simulink model "uuv_depth_control"  (R2021a)
settings: Solver=ode1  StartTime=0  StopTime=1000  FixedStep=0.1  RelTol=1e-3
undefined symbols (not defined in the file or in its folder): sigbuilder_block
(part 1 of 2)
settings Model: NumberOfSteps=10  PacingRate=1000  Creator=53549  LastModifiedBy=21847
settings DataIOCC: ReturnWorkspaceOutputs=off
settings DebuggingCC: SFMachineParentedDataDiag=warning  ArithmeticOperatorsInVariantConditions=warning
settings SFSimCC: SimUseLocalCustomCode=off  CustomCodeUndefinedFunction=UseInterfaceOnly
settings RTWCC: RTWUseLocalCustomCode=off
settings CodeAppCC: StateflowObjectComments=on

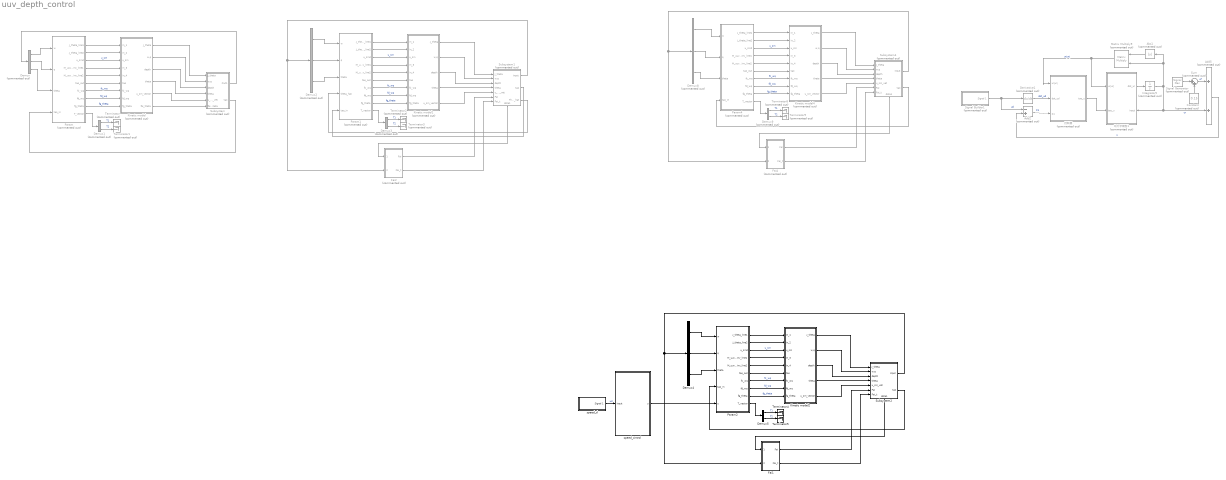
== system uuv_depth_control ==
  Abs1 : Abs  Commented=on
  Add2 : Sum  Commented=on  Inputs=-+
  Add5 : Sum  Commented=on
  Constant : Constant  Commented=on  Value=0.15
  Demux : Demux  Commented=on  Outputs=3
  Demux1 : Demux  Commented=on  Outputs=2
  Demux2 : Demux  Commented=on  Outputs=3
  Demux3 : Demux  Commented=on  Outputs=2
  Demux4 : Demux  Outputs=3
  Demux5 : Demux  Outputs=2
  Demux8 : Demux  Commented=on  Outputs=3
  Demux9 : Demux  Commented=on  Outputs=2
  Derivative1 : Derivative  Commented=on
  Fai1 : Subsystem
  Fai2 : Subsystem  Commented=on
  Fai4 : Subsystem  Commented=on
  Integrator5 : Integrator  Commented=on
  Kinetic model : Subsystem  Commented=on
  Kinetic model1 : Subsystem  Commented=on
  Kinetic model2 : Subsystem
  Kinetic model4 : Subsystem  Commented=on
  Matrix Multiply9 : Product  Commented=on  Multiplication=Matrix(*)
  Param : MATLAB Function  Commented=on  TreatAsAtomicUnit=on
  Param1 : MATLAB Function  Commented=on  TreatAsAtomicUnit=on
  Param2 : MATLAB Function  TreatAsAtomicUnit=on
  Param4 : MATLAB Function  Commented=on  TreatAsAtomicUnit=on
  Signal Generator : SignalGenerator  Commented=on  Amplitude=0.2  Frequency=0.0143
  Signal Builder1 : Subsystem  Tag=STV Subsys  Commented=on  LoadFcn=sigbuilder_block('load');  StartFcn=sigbuilder_block('start');  StopFcn=sigbuilder_block('stop');  ClipboardFcn=sigbuilder_block('clipboard');  mask(Sigbuilder block){tuvar=[0:10]}
      mask help: Simulink:masks:SigbuilderBlock_MD
      mask init:
      | if ~strcmp(get_param(bdroot(gcbh),'SimulationStatus'),'stopped') tuvar = sigbuilder_block('maskInit'); end
      settings: CopyFcn=sigbuilder_block('copy');  DeleteFcn=sigbuilder_block('delete');  ModelCloseFcn=sigbuilder_block('modelClose');  PreSaveFcn=sigbuilder_block('preSave');  PauseFcn=sigbuilder_block('pause');  ContinueFcn=sigbuilder_block('continue');  NameChangeFcn=sigbuilder_block('namechange');  OpenFcn=sigbuilder_block('open',[437.6 199.2 550.4 400 ]);  CloseFcn=sigbuilder_block('close');
      mask Display: plot(0, 0, 100, 100,[2, 2, 32, 32, 2], [68, 8, 8, 68, 68],[32, 2], [38, 38], [32, 19, 2],[53, 60, 44], [32, 17, 17, 2],[16, 16, 31, 31]);txt = getActiveGroup(gcbh);text(2, 100, txt,'verticalAlignment', 'top');
  Subsystem : Subsystem  Commented=on
  Subsystem1 : Subsystem  Commented=on
      settings: PortSchema="{\"entries\":[{\"content\":{\"sides\":[{\"content\":{\"connectorIds\":[\"In1\",\"In2\",\"In3\",\"In4\",\"In5\",\"In6\",\"In7\"]},\"type\":\"ConnectorPlacement.EquallySpacedRectSide\",\"uuid\":\"5c5a44e6-8d8e-440f-9e7c-8dc2648a5aa2\"},{\"content\":{\"connectorIds\":[\"Out1\",\"Out2\",\"Out3\"],\"side\":\"RIGHT\"},\"type\":\"ConnectorPlacement.EquallySpacedRectSide\",\"uuid\":\"bbda16c8-79bf-4e81-8c5f-170a18e1caa9\"},{\"content\":{\"connectorIds\":[],\"side\":\"TOP\"},\"type\":\"ConnectorPlacement.EquallySpacedRectSide\",\"uuid\":\"ec6df362-669b-4b04-85b5-b778e5b376fb\"},{\"content\":{\"connectorIds\":[\"Out4\"],\"side\":\"BOTTOM\"},\"type\":\"ConnectorPlacement.EquallySpacedRectSide\",\"uuid\":\"b375aecc-e755-48ed-98c2-53f6a7777844\"}]},\"type\":\"ConnectorPlacement.EquallySpacedConnector\",\"uuid\":\"a63cd60f-02eb-402d-846a-0ab9a0543d99\"}],\"packageUris\":[\"http://schema.mathworks.com/mf0/Connector/R2020b\"],\"version\":\"1.0\"}"
  Subsystem2 : Subsystem
      settings: PortSchema="{\"entries\":[{\"content\":{\"sides\":[{\"content\":{\"connectorIds\":[\"In1\",\"In2\",\"In3\",\"In4\",\"In5\",\"In6\",\"In7\"]},\"type\":\"ConnectorPlacement.EquallySpacedRectSide\",\"uuid\":\"5c5a44e6-8d8e-440f-9e7c-8dc2648a5aa2\"},{\"content\":{\"connectorIds\":[\"Out1\",\"Out2\"],\"side\":\"RIGHT\"},\"type\":\"ConnectorPlacement.EquallySpacedRectSide\",\"uuid\":\"bbda16c8-79bf-4e81-8c5f-170a18e1caa9\"},{\"content\":{\"connectorIds\":[],\"side\":\"TOP\"},\"type\":\"ConnectorPlacement.EquallySpacedRectSide\",\"uuid\":\"ec6df362-669b-4b04-85b5-b778e5b376fb\"},{\"content\":{\"connectorIds\":[\"Out3\"],\"side\":\"BOTTOM\"},\"type\":\"ConnectorPlacement.EquallySpacedRectSide\",\"uuid\":\"b375aecc-e755-48ed-98c2-53f6a7777844\"}]},\"type\":\"ConnectorPlacement.EquallySpacedConnector\",\"uuid\":\"a63cd60f-02eb-402d-846a-0ab9a0543d99\"}],\"packageUris\":[\"http://schema.mathworks.com/mf0/Connector/R2020b\"],\"version\":\"1.0\"}"
  Subsystem4 : Subsystem  Commented=on
      settings: PortSchema="{\"entries\":[{\"content\":{\"sides\":[{\"content\":{\"connectorIds\":[\"In1\",\"In2\",\"In3\",\"In4\",\"In5\",\"In6\",\"In7\"]},\"type\":\"ConnectorPlacement.EquallySpacedRectSide\",\"uuid\":\"5c5a44e6-8d8e-440f-9e7c-8dc2648a5aa2\"},{\"content\":{\"connectorIds\":[\"Out1\",\"Out2\"],\"side\":\"RIGHT\"},\"type\":\"ConnectorPlacement.EquallySpacedRectSide\",\"uuid\":\"bbda16c8-79bf-4e81-8c5f-170a18e1caa9\"},{\"content\":{\"connectorIds\":[],\"side\":\"TOP\"},\"type\":\"ConnectorPlacement.EquallySpacedRectSide\",\"uuid\":\"ec6df362-669b-4b04-85b5-b778e5b376fb\"},{\"content\":{\"connectorIds\":[\"Out3\"],\"side\":\"BOTTOM\"},\"type\":\"ConnectorPlacement.EquallySpacedRectSide\",\"uuid\":\"b375aecc-e755-48ed-98c2-53f6a7777844\"}]},\"type\":\"ConnectorPlacement.EquallySpacedConnector\",\"uuid\":\"a63cd60f-02eb-402d-846a-0ab9a0543d99\"}],\"packageUris\":[\"http://schema.mathworks.com/mf0/Connector/R2020b\"],\"version\":\"1.0\"}"
  Sum : Sum  Commented=on  Inputs=|++
  Terminator{,1..3,8..9} (6 alike) : Terminator  Commented=on
  Terminator4 : Terminator
  Terminator5 : Terminator
  speed_cintrol : Subsystem
  speed_d : Subsystem  Tag=STV Subsys  LoadFcn=sigbuilder_block('load');  StartFcn=sigbuilder_block('start');  StopFcn=sigbuilder_block('stop');  ClipboardFcn=sigbuilder_block('clipboard');  mask(Sigbuilder block){tuvar=[0:10]}
      mask help: Simulink:masks:SigbuilderBlock_MD
      mask init:
      | if ~strcmp(get_param(bdroot(gcbh),'SimulationStatus'),'stopped') tuvar = sigbuilder_block('maskInit'); end
      settings: CopyFcn=sigbuilder_block('copy');  DeleteFcn=sigbuilder_block('delete');  ModelCloseFcn=sigbuilder_block('modelClose');  PreSaveFcn=sigbuilder_block('preSave');  PauseFcn=sigbuilder_block('pause');  ContinueFcn=sigbuilder_block('continue');  NameChangeFcn=sigbuilder_block('namechange');  OpenFcn=sigbuilder_block('open',[437.6 199.2 550.4 400 ]);  CloseFcn=sigbuilder_block('close');
      mask Display: plot(0, 0, 100, 100,[2, 2, 32, 32, 2], [68, 8, 8, 68, 68],[32, 2], [38, 38], [32, 19, 2],[53, 60, 44], [32, 17, 17, 2],[16, 16, 31, 31]);txt = getActiveGroup(gcbh);text(2, 100, txt,'verticalAlignment', 'top');
  动力学模型1 : Subsystem  Commented=on
      settings: PortSchema="{\"entries\":[{\"content\":{\"sides\":[{\"content\":{\"connectorIds\":[\"In1\",\"In2\"]},\"type\":\"ConnectorPlacement.EquallySpacedRectSide\",\"uuid\":\"ab557843-e031-4248-b9d1-7c566f741c61\"},{\"content\":{\"connectorIds\":[\"Out1\",\"In3\"],\"side\":\"RIGHT\"},\"type\":\"ConnectorPlacement.EquallySpacedRectSide\",\"uuid\":\"21457043-a342-42ad-b992-fc1f26888830\"},{\"content\":{\"connectorIds\":[],\"side\":\"TOP\"},\"type\":\"ConnectorPlacement.EquallySpacedRectSide\",\"uuid\":\"46297411-6c48-4449-b379-31c60e59c869\"}]},\"type\":\"ConnectorPlacement.EquallySpacedConnector\",\"uuid\":\"5361bacf-5f38-4767-97c2-c3369bc5e695\"}],\"packageUris\":[\"http://schema.mathworks.com/mf0/Connector/R2020b\"],\"version\":\"1.0\"}"
  控制器 : Subsystem  Commented=on
  wires:
  Demux/1 -> Param/1(w)
  Demux/2 -> Param/2(q)
  Demux/3 -> Param/3(theta)
  Param/1(J_theta_line1) -> Kinetic model/1(in_1)
  Param/2(J_theta_line2) -> Kinetic model/2(in_2)
  Param/3(u_sind) -> Kinetic model/3(u_sin)  "u_sin"
  Param/4(M_uuv_inv_line1) -> Kinetic model/4(in_3)
  Param/5(M_uuv_inv_line2) -> Kinetic model/5(in_4)
  Param/7(fc_wq) -> Kinetic model/7(fc_wq)  "fc_wq"
  Param/8(fd_wq) -> Kinetic model/8(fd_wq)  "fd_wq"
  Param/9(fg_theta) -> Kinetic model/9(fg_theta)  "fg_theta"
  Kinetic model/1(J_theta) -> Subsystem/1(J_theta)
  Kinetic model/2(w,q) -> Subsystem/2(w;q)
  Kinetic model/3(depth) -> Subsystem/3(depth)
  Kinetic model/4(theta) -> Subsystem/4(theta)
  Kinetic model/5(u_sin_vector) -> Subsystem/5(u_sin_vet)
  Kinetic model/6(fai_theta) -> Subsystem/6(fai_theta)
  Subsystem/1(Out1) -> Demux/1
  Subsystem/2(tao) -> Param/4(tao_in)
  Param/10(T_vector) -> Demux1/1
  Demux1/1 -> Terminator/1  "T1"
  Demux1/2 -> Terminator1/1  "T2"
  Param/6(tao_out) -> Kinetic model/6(tao)
  Param1/2(J_theta_line2) -> Kinetic model1/2(in_2)
  Param1/10(T_vector) -> Demux3/1
  Demux2/1 -> Param1/1(w)
  Demux2/3 -> Param1/3(theta)
  Param1/4(M_uuv_inv_line1) -> Kinetic model1/4(in_3)
  Kinetic model1/2(w,q) -> Subsystem1/2(w;q)
  Subsystem1/1(Input) -> Demux2/1, Fai2/2(Input)
  Param1/9(fg_theta) -> Kinetic model1/9(fg_theta)  "fg_theta"
  Param1/3(u_sind) -> Kinetic model1/3(u_sin)  "u_sin"
  Demux2/2 -> Param1/2(q)
  Demux3/1 -> Terminator2/1  "T1"
  Param1/8(fd_wq) -> Kinetic model1/8(fd_wq)  "fd_wq"
  Param1/7(fc_wq) -> Kinetic model1/7(fc_wq)  "fc_wq"
  Kinetic model1/1(J_theta) -> Subsystem1/1(J_theta)
  Param1/1(J_theta_line1) -> Kinetic model1/1(in_1)
  Kinetic model1/3(depth) -> Subsystem1/3(depth)
  Param1/6(tao_out) -> Kinetic model1/6(tao)
  Kinetic model1/4(theta) -> Subsystem1/4(theta)
  Fai2/1(Fai) -> Subsystem1/6(Fai)
  Demux3/2 -> Terminator3/1  "T2"
  Kinetic model1/5(u_sin_vector) -> Subsystem1/5(u_sin_vet)
  Fai2/2(Fai_t) -> Subsystem1/7(Fai_t)
  Param1/5(M_uuv_inv_line2) -> Kinetic model1/5(in_4)
  Subsystem1/3(Theta_hat) -> Param1/4(theta_hat)
  Subsystem1/2(tao) -> Param1/5(tao_in)
  Subsystem1/4(dota1) -> Fai2/1(dota1)
  Fai4/2(Fai_t) -> Subsystem4/7(Fai_t)
  Subsystem4/3(dota1) -> Fai4/1(dota1)
  Demux8/2 -> Param4/2(q)
  Subsystem4/1(Input) -> Demux8/1, Fai4/2(Input)
  Demux9/2 -> Terminator9/1  "T2"
  Kinetic model4/5(u_sin_vector) -> Subsystem4/5(u_sin_vet)
  Fai4/1(Fai) -> Subsystem4/6(Fai)
  Param4/5(M_uuv_inv_line2) -> Kinetic model4/5(in_4)
  Param4/8(fd_wq) -> Kinetic model4/8(fd_wq)  "fd_wq"
  Kinetic model4/4(theta) -> Subsystem4/4(theta)
  Param4/7(fc_wq) -> Kinetic model4/7(fc_wq)  "fc_wq"
  Param4/6(tao_out) -> Kinetic model4/6(tao)
  Subsystem4/2(tao) -> Param4/4(tao_in)
  Kinetic model4/3(depth) -> Subsystem4/3(depth)
  Demux8/1 -> Param4/1(w)
  Param4/9(fg_theta) -> Kinetic model4/9(fg_theta)  "fg_theta"
  Demux9/1 -> Terminator8/1  "T1"
  Kinetic model4/2(w,q) -> Subsystem4/2(w;q)
  Param4/1(J_theta_line1) -> Kinetic model4/1(in_1)
  Demux8/3 -> Param4/3(theta)
  Param4/4(M_uuv_inv_line1) -> Kinetic model4/4(in_3)
  Param4/10(T_vector) -> Demux9/1
  Param4/3(u_sind) -> Kinetic model4/3(u_sin)  "u_sin"
  Kinetic model4/1(J_theta) -> Subsystem4/1(J_theta)
  Param4/2(J_theta_line2) -> Kinetic model4/2(in_2)
  Param2/3(u_sind) -> Kinetic model2/3(u_sin)  "u_sin"
  Param2/2(J_theta_line2) -> Kinetic model2/2(in_2)
  Param2/4(M_uuv_inv_line1) -> Kinetic model2/4(in_3)
  Param2/1(J_theta_line1) -> Kinetic model2/1(in_1)
  Demux4/3 -> Param2/3(theta)
  Kinetic model2/2(w,q) -> Subsystem2/2(w;q)
  Param2/9(fg_theta) -> Kinetic model2/9(fg_theta)  "fg_theta"
  Param2/7(fc_wq) -> Kinetic model2/7(fc_wq)  "fc_wq"
  Kinetic model2/3(depth) -> Subsystem2/3(depth)
  Param2/6(tao_out) -> Kinetic model2/6(tao)
  Subsystem2/2(tao) -> Param2/4(tao_in)
  Param2/5(M_uuv_inv_line2) -> Kinetic model2/5(in_4)
  Kinetic model2/1(J_theta) -> Subsystem2/1(J_theta)
  Param2/8(fd_wq) -> Kinetic model2/8(fd_wq)  "fd_wq"
  Fai1/1(Fai) -> Subsystem2/6(Fai)
  Demux5/1 -> Terminator4/1  "T1"
  Kinetic model2/4(theta) -> Subsystem2/4(theta)
  Demux4/1 -> Param2/1(w)
  Subsystem2/3(dota1) -> Fai1/1(dota1)
  Subsystem2/1(Input) -> Demux4/1, Fai1/2(Input)
  Demux4/2 -> Param2/2(q)
  Demux5/2 -> Terminator5/1  "T2"
  Kinetic model2/5(u_sin_vector) -> Subsystem2/5(u_sin_vet)
  Param2/10(T_vector) -> Demux5/1
  Fai1/2(Fai_t) -> Subsystem2/7(Fai_t)
  Signal Generator/1 -> Sum/1
  Signal Builder1/1(Signal 1) -> Add2/1, Derivative1/1  "ud"
  Constant/1 -> Sum/2
  控制器/1(tao_u) -> 动力学模型1/2(tao_u)
  Sum/1 -> Add5/1  "uf"
  Abs1/1 -> Matrix Multiply9/1
  Derivative1/1 -> 控制器/2(dot_ud)  "dot_ud"
  Integrator5/1 -> 动力学模型1/3(Input), Add5/2, Matrix Multiply9/2, Abs1/1  "ur"
  动力学模型1/1(dot_ur) -> Integrator5/1
  Add2/1 -> 控制器/3(Z1)  "Z1"
  Add5/1 -> Add2/2  "u"
  Matrix Multiply9/1 -> 控制器/1(ur|ur|), 动力学模型1/1(ur|ur|)  "ur|ur|"
  speed_cintrol/1(u) -> Param2/5(u)
  speed_d/1(Signal 1) -> speed_cintrol/1(Input)  "ud"

== system uuv_depth_control/Fai1 ==
  dota1 : Inport
  Input : Inport  Port=2
  Abs : Abs
  Abs1 : Abs
  Demux : Demux  Outputs=3
  Demux1 : Demux  Outputs=2
  MATLAB Function : MATLAB Function  TreatAsAtomicUnit=on
  Matrix Multiply : Product  Multiplication=Matrix(*)
  Matrix Multiply1 : Product  Multiplication=Matrix(*)
  Matrix Multiply2 : Product  Multiplication=Matrix(*)
  Square : Math  Operator=square  SaturateOnIntegerOverflow=on
  Fai : Outport
  Fai_t : Outport  Port=2
  wires:
  Input/1 -> Demux/1
  Demux/1 -> Matrix Multiply2/2, Abs/1, MATLAB Function/2(w), Matrix Multiply/2  "w"
  Demux/3 -> MATLAB Function/9(theta)  "theta"
  Abs/1 -> Matrix Multiply/1
  Matrix Multiply/1 -> MATLAB Function/1(w_w_)  "w|w|"
  Abs1/1 -> Matrix Multiply1/1
  Demux/2 -> Abs1/1, Matrix Multiply1/2, MATLAB Function/5(q), Matrix Multiply2/1, Square/1  "q"
  Matrix Multiply1/1 -> MATLAB Function/4(q_q_)  "q|q|"
  Square/1 -> MATLAB Function/7(q_2)  "q^2"
  Matrix Multiply2/1 -> MATLAB Function/8(wq)  "wq"
  MATLAB Function/1(Fai) -> Fai/1
  MATLAB Function/2(Fai_t) -> Fai_t/1
  dota1/1 -> Demux1/1
  Demux1/1 -> MATLAB Function/3(dotw)
  Demux1/2 -> MATLAB Function/6(dotq)

== system uuv_depth_control/Fai2 ==
  dota1 : Inport
  Input : Inport  Port=2
  Abs : Abs
  Abs1 : Abs
  Demux : Demux  Outputs=3
  Demux1 : Demux  Outputs=2
  MATLAB Function : MATLAB Function  TreatAsAtomicUnit=on
  Matrix Multiply : Product  Multiplication=Matrix(*)
  Matrix Multiply1 : Product  Multiplication=Matrix(*)
  Matrix Multiply2 : Product  Multiplication=Matrix(*)
  Square : Math  Operator=square  SaturateOnIntegerOverflow=on
  Fai : Outport
  Fai_t : Outport  Port=2
  wires:
  Input/1 -> Demux/1
  Demux/1 -> Matrix Multiply2/2, Abs/1, MATLAB Function/2(w), Matrix Multiply/2  "w"
  Demux/3 -> MATLAB Function/9(theta)  "theta"
  Abs/1 -> Matrix Multiply/1
  Matrix Multiply/1 -> MATLAB Function/1(w_w_)  "w|w|"
  Abs1/1 -> Matrix Multiply1/1
  Demux/2 -> Abs1/1, Matrix Multiply1/2, MATLAB Function/5(q), Matrix Multiply2/1, Square/1  "q"
  Matrix Multiply1/1 -> MATLAB Function/4(q_q_)  "q|q|"
  Square/1 -> MATLAB Function/7(q_2)  "q^2"
  Matrix Multiply2/1 -> MATLAB Function/8(wq)  "wq"
  MATLAB Function/1(Fai) -> Fai/1
  MATLAB Function/2(Fai_t) -> Fai_t/1
  dota1/1 -> Demux1/1
  Demux1/1 -> MATLAB Function/3(dotw)
  Demux1/2 -> MATLAB Function/6(dotq)

== system uuv_depth_control/Fai4 ==
  dota1 : Inport
  Input : Inport  Port=2
  Abs : Abs
  Abs1 : Abs
  Demux : Demux  Outputs=3
  Demux1 : Demux  Outputs=2
  MATLAB Function : MATLAB Function  TreatAsAtomicUnit=on
  Matrix Multiply : Product  Multiplication=Matrix(*)
  Matrix Multiply1 : Product  Multiplication=Matrix(*)
  Matrix Multiply2 : Product  Multiplication=Matrix(*)
  Square : Math  Operator=square  SaturateOnIntegerOverflow=on
  Fai : Outport
  Fai_t : Outport  Port=2
  wires:
  Input/1 -> Demux/1
  Demux/1 -> Matrix Multiply2/2, Abs/1, MATLAB Function/2(w), Matrix Multiply/2  "w"
  Demux/3 -> MATLAB Function/9(theta)  "theta"
  Abs/1 -> Matrix Multiply/1
  Matrix Multiply/1 -> MATLAB Function/1(w_w_)  "w|w|"
  Abs1/1 -> Matrix Multiply1/1
  Demux/2 -> Abs1/1, Matrix Multiply1/2, MATLAB Function/5(q), Matrix Multiply2/1, Square/1  "q"
  Matrix Multiply1/1 -> MATLAB Function/4(q_q_)  "q|q|"
  Square/1 -> MATLAB Function/7(q_2)  "q^2"
  Matrix Multiply2/1 -> MATLAB Function/8(wq)  "wq"
  MATLAB Function/1(Fai) -> Fai/1
  MATLAB Function/2(Fai_t) -> Fai_t/1
  dota1/1 -> Demux1/1
  Demux1/1 -> MATLAB Function/3(dotw)
  Demux1/2 -> MATLAB Function/6(dotq)

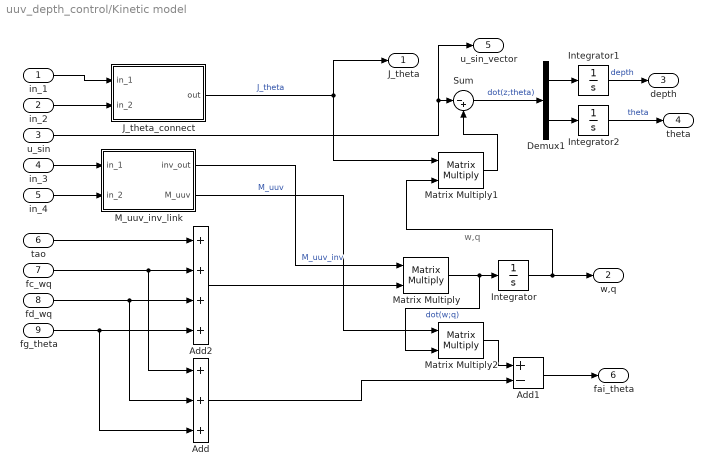
== system uuv_depth_control/Kinetic model ==
  note: w,q
  in_1 : Inport
  in_2 : Inport  Port=2
  u_sin : Inport  Port=3
  in_3 : Inport  Port=4
  in_4 : Inport  Port=5
  tao : Inport  Port=6
  fc_wq : Inport  Port=7
  fd_wq : Inport  Port=8
  fg_theta : Inport  Port=9
  Add : Sum  Inputs=+++
  Add1 : Sum  Inputs=+-
  Add2 : Sum  Inputs=++++
  Demux1 : Demux  Outputs=2
  Integrator : Integrator
  Integrator1 : Integrator
  Integrator2 : Integrator
  J_theta_connect : MATLAB Function  TreatAsAtomicUnit=on
  M_uuv_inv_link : MATLAB Function  TreatAsAtomicUnit=on
  Matrix Multiply : Product  Multiplication=Matrix(*)
  Matrix Multiply1 : Product  Multiplication=Matrix(*)
  Matrix Multiply2 : Product  Multiplication=Matrix(*)
  Sum : Sum  Inputs=|-+
  J_theta : Outport
  w,q : Outport  Port=2
  depth : Outport  Port=3
  theta : Outport  Port=4
  u_sin_vector : Outport  Port=5
  fai_theta : Outport  Port=6
  wires:
  Matrix Multiply/1 -> Matrix Multiply2/2, Integrator/1  "dot(w;q)"
  Sum/1 -> Demux1/1  "dot(z;theta)"
  Add2/1 -> Matrix Multiply/2
  Integrator/1 -> w,q/1, Matrix Multiply1/2
  u_sin/1 -> u_sin_vector/1, Sum/1
  Matrix Multiply1/1 -> Sum/2
  M_uuv_inv_link/1(inv_out) -> Matrix Multiply/1  "M_uuv_inv"
  J_theta_connect/1(out) -> J_theta/1, Matrix Multiply1/1  "J_theta"
  in_2/1 -> J_theta_connect/2(in_2)
  in_1/1 -> J_theta_connect/1(in_1)
  in_3/1 -> M_uuv_inv_link/1(in_1)
  in_4/1 -> M_uuv_inv_link/2(in_2)
  Integrator1/1 -> depth/1  "depth"
  Demux1/1 -> Integrator1/1
  Demux1/2 -> Integrator2/1
  Integrator2/1 -> theta/1  "theta"
  M_uuv_inv_link/2(M_uuv) -> Matrix Multiply2/1  "M_uuv"
  Matrix Multiply2/1 -> Add1/1
  Add1/1 -> fai_theta/1
  tao/1 -> Add2/1
  fc_wq/1 -> Add/1, Add2/2
  fd_wq/1 -> Add/2, Add2/3
  fg_theta/1 -> Add/3, Add2/4
  Add/1 -> Add1/2

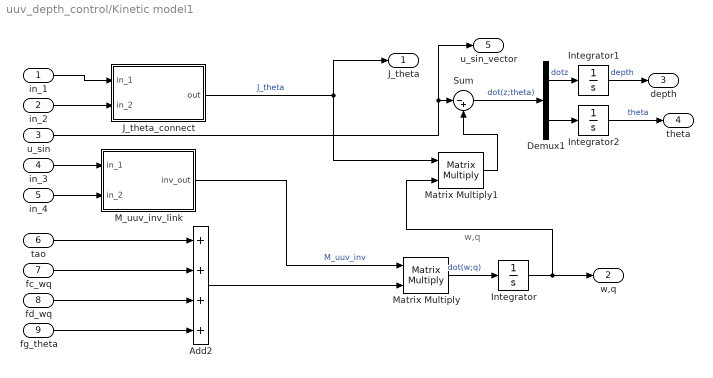
== system uuv_depth_control/Kinetic model1 ==
  note: w,q
  in_1 : Inport
  in_2 : Inport  Port=2
  u_sin : Inport  Port=3
  in_3 : Inport  Port=4
  in_4 : Inport  Port=5
  tao : Inport  Port=6
  fc_wq : Inport  Port=7
  fd_wq : Inport  Port=8
  fg_theta : Inport  Port=9
  Add2 : Sum  Inputs=++++
  Demux1 : Demux  Outputs=2
  Integrator : Integrator
  Integrator1 : Integrator
  Integrator2 : Integrator
  J_theta_connect : MATLAB Function  TreatAsAtomicUnit=on
  M_uuv_inv_link : MATLAB Function  TreatAsAtomicUnit=on
  Matrix Multiply : Product  Multiplication=Matrix(*)
  Matrix Multiply1 : Product  Multiplication=Matrix(*)
  Sum : Sum  Inputs=|-+
  J_theta : Outport
  w,q : Outport  Port=2
  depth : Outport  Port=3
  theta : Outport  Port=4
  u_sin_vector : Outport  Port=5
  wires:
  Matrix Multiply/1 -> Integrator/1  "dot(w;q)"
  Sum/1 -> Demux1/1  "dot(z;theta)"
  Add2/1 -> Matrix Multiply/2
  Integrator/1 -> w,q/1, Matrix Multiply1/2
  u_sin/1 -> u_sin_vector/1, Sum/1
  Matrix Multiply1/1 -> Sum/2
  M_uuv_inv_link/1(inv_out) -> Matrix Multiply/1  "M_uuv_inv"
  J_theta_connect/1(out) -> J_theta/1, Matrix Multiply1/1  "J_theta"
  in_2/1 -> J_theta_connect/2(in_2)
  in_1/1 -> J_theta_connect/1(in_1)
  in_3/1 -> M_uuv_inv_link/1(in_1)
  in_4/1 -> M_uuv_inv_link/2(in_2)
  Integrator1/1 -> depth/1  "depth"
  Demux1/1 -> Integrator1/1  "dotz"
  Demux1/2 -> Integrator2/1
  Integrator2/1 -> theta/1  "theta"
  tao/1 -> Add2/1
  fc_wq/1 -> Add2/2
  fd_wq/1 -> Add2/3
  fg_theta/1 -> Add2/4

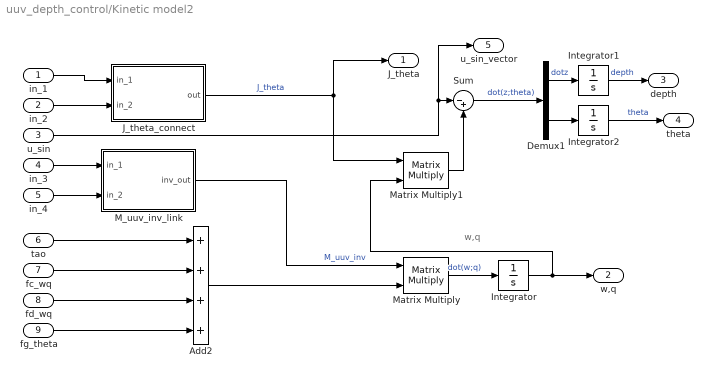
== system uuv_depth_control/Kinetic model2 ==
  note: w,q
  in_1 : Inport
  in_2 : Inport  Port=2
  u_sin : Inport  Port=3
  in_3 : Inport  Port=4
  in_4 : Inport  Port=5
  tao : Inport  Port=6
  fc_wq : Inport  Port=7
  fd_wq : Inport  Port=8
  fg_theta : Inport  Port=9
  Add2 : Sum  Inputs=++++
  Demux1 : Demux  Outputs=2
  Integrator : Integrator
  Integrator1 : Integrator
  Integrator2 : Integrator
  J_theta_connect : MATLAB Function  TreatAsAtomicUnit=on
  M_uuv_inv_link : MATLAB Function  TreatAsAtomicUnit=on
  Matrix Multiply : Product  Multiplication=Matrix(*)
  Matrix Multiply1 : Product  Multiplication=Matrix(*)
  Sum : Sum  Inputs=|-+
  J_theta : Outport
  w,q : Outport  Port=2
  depth : Outport  Port=3
  theta : Outport  Port=4
  u_sin_vector : Outport  Port=5
  wires:
  Matrix Multiply/1 -> Integrator/1  "dot(w;q)"
  Sum/1 -> Demux1/1  "dot(z;theta)"
  Add2/1 -> Matrix Multiply/2
  Integrator/1 -> w,q/1, Matrix Multiply1/2
  u_sin/1 -> u_sin_vector/1, Sum/1
  Matrix Multiply1/1 -> Sum/2
  M_uuv_inv_link/1(inv_out) -> Matrix Multiply/1  "M_uuv_inv"
  J_theta_connect/1(out) -> J_theta/1, Matrix Multiply1/1  "J_theta"
  in_2/1 -> J_theta_connect/2(in_2)
  in_1/1 -> J_theta_connect/1(in_1)
  in_3/1 -> M_uuv_inv_link/1(in_1)
  in_4/1 -> M_uuv_inv_link/2(in_2)
  Integrator1/1 -> depth/1  "depth"
  Demux1/1 -> Integrator1/1  "dotz"
  Demux1/2 -> Integrator2/1
  Integrator2/1 -> theta/1  "theta"
  tao/1 -> Add2/1
  fc_wq/1 -> Add2/2
  fd_wq/1 -> Add2/3
  fg_theta/1 -> Add2/4

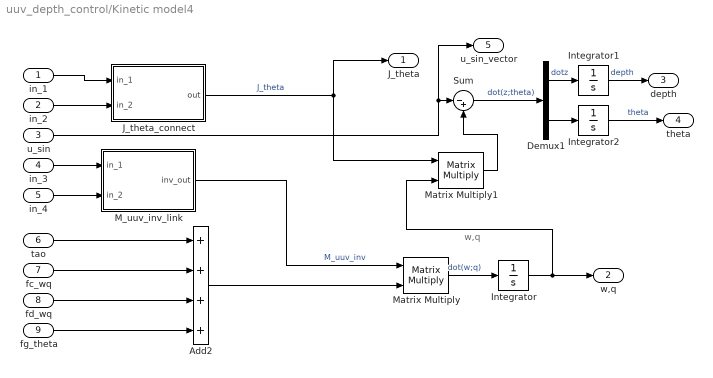
== system uuv_depth_control/Kinetic model4 ==
  note: w,q
  in_1 : Inport
  in_2 : Inport  Port=2
  u_sin : Inport  Port=3
  in_3 : Inport  Port=4
  in_4 : Inport  Port=5
  tao : Inport  Port=6
  fc_wq : Inport  Port=7
  fd_wq : Inport  Port=8
  fg_theta : Inport  Port=9
  Add2 : Sum  Inputs=++++
  Demux1 : Demux  Outputs=2
  Integrator : Integrator
  Integrator1 : Integrator
  Integrator2 : Integrator
  J_theta_connect : MATLAB Function  TreatAsAtomicUnit=on
  M_uuv_inv_link : MATLAB Function  TreatAsAtomicUnit=on
  Matrix Multiply : Product  Multiplication=Matrix(*)
  Matrix Multiply1 : Product  Multiplication=Matrix(*)
  Sum : Sum  Inputs=|-+
  J_theta : Outport
  w,q : Outport  Port=2
  depth : Outport  Port=3
  theta : Outport  Port=4
  u_sin_vector : Outport  Port=5
  wires:
  Matrix Multiply/1 -> Integrator/1  "dot(w;q)"
  Sum/1 -> Demux1/1  "dot(z;theta)"
  Add2/1 -> Matrix Multiply/2
  Integrator/1 -> w,q/1, Matrix Multiply1/2
  u_sin/1 -> u_sin_vector/1, Sum/1
  Matrix Multiply1/1 -> Sum/2
  M_uuv_inv_link/1(inv_out) -> Matrix Multiply/1  "M_uuv_inv"
  J_theta_connect/1(out) -> J_theta/1, Matrix Multiply1/1  "J_theta"
  in_2/1 -> J_theta_connect/2(in_2)
  in_1/1 -> J_theta_connect/1(in_1)
  in_3/1 -> M_uuv_inv_link/1(in_1)
  in_4/1 -> M_uuv_inv_link/2(in_2)
  Integrator1/1 -> depth/1  "depth"
  Demux1/1 -> Integrator1/1  "dotz"
  Demux1/2 -> Integrator2/1
  Integrator2/1 -> theta/1  "theta"
  tao/1 -> Add2/1
  fc_wq/1 -> Add2/2
  fd_wq/1 -> Add2/3
  fg_theta/1 -> Add2/4

== system uuv_depth_control/Signal Builder1 ==
  Demux : Demux  Tag=STV Demux  Outputs=1
      settings: DisplayOption=none
  FromWs : FromWorkspace  Tag=STV FromWs  VariableName=tuvar
      SigBuilderData=|
      | common.afterFinalStr = 'Extrapolate'
      | common.sampleTime = 0
      | dataSet.timeRange = [0 10]
      | dataSet.name = 'Group 1'
      | sbobj.Groups.Name = 'Group 1'
      | sbobj.Groups.Signals.Name = 'Signal 1'
      | sbobj.Groups.Signals.XData = [0 10]
      | sbobj.Groups.Signals.YData = [1.2 1.2]
  Signal 1 : Outport  Tag=STV Outport
  wires:
  FromWs/1 -> Demux/1
  Demux/1 -> Signal 1/1

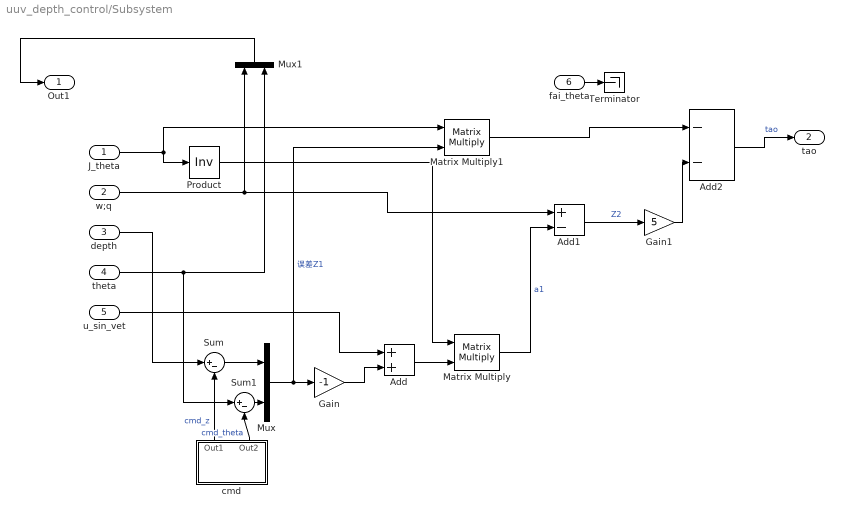
== system uuv_depth_control/Subsystem ==
  J_theta : Inport
  w;q : Inport  Port=2
  depth : Inport  Port=3
  theta : Inport  Port=4
  u_sin_vet : Inport  Port=5
  fai_theta : Inport  Port=6
  Add : Sum
  Add1 : Sum  Inputs=+-
  Add2 : Sum  Inputs=--
  Gain : Gain  Gain=-1
  Gain1 : Gain  Gain=5
  Matrix Multiply : Product  Multiplication=Matrix(*)
  Matrix Multiply1 : Product  Multiplication=Matrix(*)
  Mux : Mux  Inputs=2
  Mux1 : Mux  Inputs=2
  Product : Product  Inputs=/  Multiplication=Matrix(*)
  Sum : Sum  Inputs=|+-
  Sum1 : Sum  Inputs=|+-
  Terminator : Terminator
  cmd : Subsystem
  Out1 : Outport
  tao : Outport  Port=2
  wires:
  Matrix Multiply/1 -> Add1/2  "a1"
  Add2/1 -> tao/1  "tao"
  Add/1 -> Matrix Multiply/2
  cmd/1(Out1) -> Sum/2  "cmd_z"
  Add1/1 -> Gain1/1  "Z2"
  Mux/1 -> Matrix Multiply1/2, Gain/1  "误差Z1"
  J_theta/1 -> Product/1, Matrix Multiply1/1
  Sum1/1 -> Mux/2
  Sum/1 -> Mux/1
  Gain/1 -> Add/2
  theta/1 -> Sum1/1, Mux1/2
  cmd/2(Out2) -> Sum1/2  "cmd_theta"
  Product/1 -> Matrix Multiply/1
  Matrix Multiply1/1 -> Add2/1
  w;q/1 -> Add1/1, Mux1/1
  depth/1 -> Sum/1
  u_sin_vet/1 -> Add/1
  Mux1/1 -> Out1/1
  Gain1/1 -> Add2/2
  fai_theta/1 -> Terminator/1

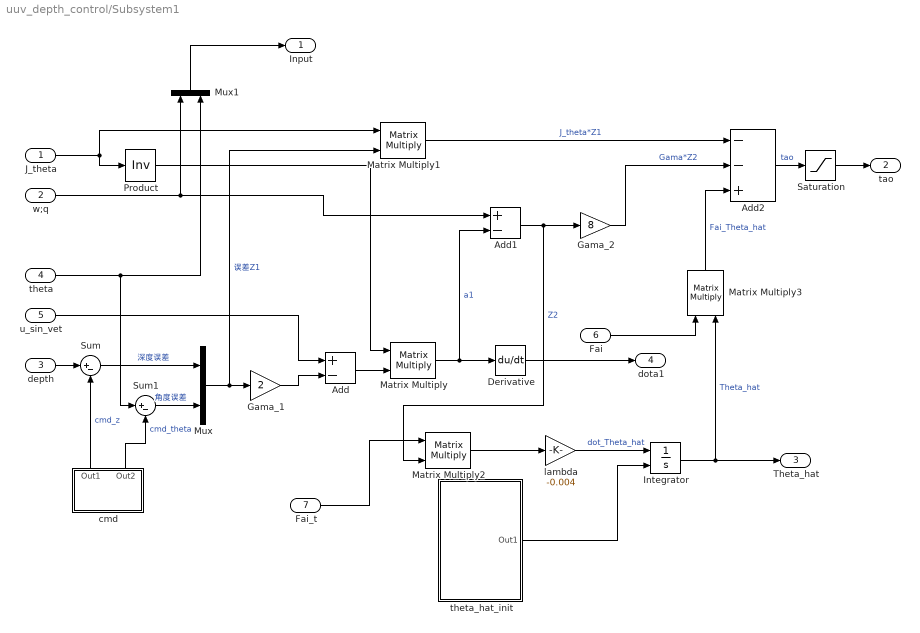
== system uuv_depth_control/Subsystem1 ==
  J_theta : Inport
  w;q : Inport  Port=2
  depth : Inport  Port=3
  theta : Inport  Port=4
  u_sin_vet : Inport  Port=5
  Fai : Inport  Port=6
  Fai_t : Inport  Port=7
  Add : Sum  Inputs=+-
  Add1 : Sum  Inputs=+-
  Add2 : Sum  Inputs=--+
  Derivative : Derivative
  Gama_1 : Gain  Gain=2
  Gama_2 : Gain  Gain=8
  Integrator : Integrator  InitialConditionSource=external
  Matrix Multiply{,1..3} (4 alike) : Product  Multiplication=Matrix(*)
  Mux : Mux  Inputs=2
  Mux1 : Mux  Inputs=2
  Product : Product  Inputs=/  Multiplication=Matrix(*)
  Saturation : Saturate  UpperLimit=120  LowerLimit=-100
  Sum : Sum  Inputs=|+-
  Sum1 : Sum  Inputs=|+-
  cmd : Subsystem
  lambda : Gain  Gain=-0.004
  theta_hat_init : Subsystem
  Input : Outport
  tao : Outport  Port=2
  Theta_hat : Outport  Port=3
  dota1 : Outport  Port=4
  wires:
  Matrix Multiply/1 -> Add1/2, Derivative/1  "a1"
  Add2/1 -> Saturation/1  "tao"
  Add/1 -> Matrix Multiply/2
  cmd/1(Out1) -> Sum/2  "cmd_z"
  Add1/1 -> Gama_2/1, Matrix Multiply2/2  "Z2"
  Mux/1 -> Matrix Multiply1/2, Gama_1/1  "误差Z1"
  J_theta/1 -> Product/1, Matrix Multiply1/1
  Sum1/1 -> Mux/2  "角度误差"
  Gama_1/1 -> Add/2
  theta/1 -> Mux1/2, Sum1/1
  cmd/2(Out2) -> Sum1/2  "cmd_theta"
  Product/1 -> Matrix Multiply/1
  Matrix Multiply1/1 -> Add2/1  "J_theta*Z1"
  w;q/1 -> Add1/1, Mux1/1
  depth/1 -> Sum/1
  u_sin_vet/1 -> Add/1
  Mux1/1 -> Input/1
  Gama_2/1 -> Add2/2  "Gama*Z2"
  Matrix Multiply2/1 -> lambda/1
  Fai_t/1 -> Matrix Multiply2/1
  Fai/1 -> Matrix Multiply3/1
  Matrix Multiply3/1 -> Add2/3  "Fai_Theta_hat"
  Integrator/1 -> Theta_hat/1, Matrix Multiply3/2  "Theta_hat"
  theta_hat_init/1(Out1) -> Integrator/2
  lambda/1 -> Integrator/1  "dot_Theta_hat"
  Derivative/1 -> dota1/1
  Sum/1 -> Mux/1  "深度误差"
  Saturation/1 -> tao/1

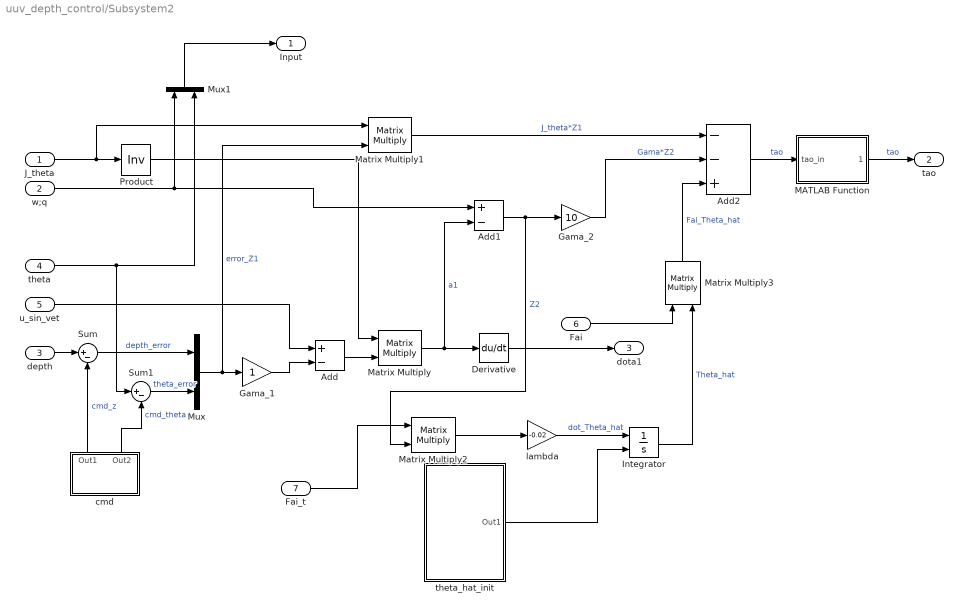
== system uuv_depth_control/Subsystem2 ==
  J_theta : Inport
  w;q : Inport  Port=2
  depth : Inport  Port=3
  theta : Inport  Port=4
  u_sin_vet : Inport  Port=5
  Fai : Inport  Port=6
  Fai_t : Inport  Port=7
  Add : Sum  Inputs=+-
  Add1 : Sum  Inputs=+-
  Add2 : Sum  Inputs=--+
  Derivative : Derivative
  Gama_1 : Gain
  Gama_2 : Gain  Gain=10
  Integrator : Integrator  InitialConditionSource=external
  MATLAB Function : MATLAB Function  TreatAsAtomicUnit=on
  Matrix Multiply{,1..3} (4 alike) : Product  Multiplication=Matrix(*)
  Mux : Mux  Inputs=2
  Mux1 : Mux  Inputs=2
  Product : Product  Inputs=/  Multiplication=Matrix(*)
  Sum : Sum  Inputs=|+-
  Sum1 : Sum  Inputs=|+-
  cmd : Subsystem
  lambda : Gain  Gain=-0.02
  theta_hat_init : Subsystem
  Input : Outport
  tao : Outport  Port=2
  dota1 : Outport  Port=3
  wires:
  Matrix Multiply/1 -> Add1/2, Derivative/1  "a1"
  Add2/1 -> MATLAB Function/1(tao_in)  "tao"
  Add/1 -> Matrix Multiply/2
  cmd/1(Out1) -> Sum/2  "cmd_z"
  Add1/1 -> Gama_2/1, Matrix Multiply2/2  "Z2"
  Mux/1 -> Matrix Multiply1/2, Gama_1/1  "error_Z1"
  J_theta/1 -> Matrix Multiply1/1, Product/1
  Sum1/1 -> Mux/2  "theta_error"
  Gama_1/1 -> Add/2
  theta/1 -> Mux1/2, Sum1/1
  cmd/2(Out2) -> Sum1/2  "cmd_theta"
  Product/1 -> Matrix Multiply/1
  Matrix Multiply1/1 -> Add2/1  "J_theta*Z1"
  w;q/1 -> Add1/1, Mux1/1
  depth/1 -> Sum/1
  u_sin_vet/1 -> Add/1
  Mux1/1 -> Input/1
  Gama_2/1 -> Add2/2  "Gama*Z2"
  Matrix Multiply2/1 -> lambda/1
  Fai_t/1 -> Matrix Multiply2/1
  Fai/1 -> Matrix Multiply3/1
  Matrix Multiply3/1 -> Add2/3  "Fai_Theta_hat"
  Integrator/1 -> Matrix Multiply3/2  "Theta_hat"
  theta_hat_init/1(Out1) -> Integrator/2
  lambda/1 -> Integrator/1  "dot_Theta_hat"
  Derivative/1 -> dota1/1
  Sum/1 -> Mux/1  "depth_error"
  MATLAB Function/1(tao_out) -> tao/1  "tao"

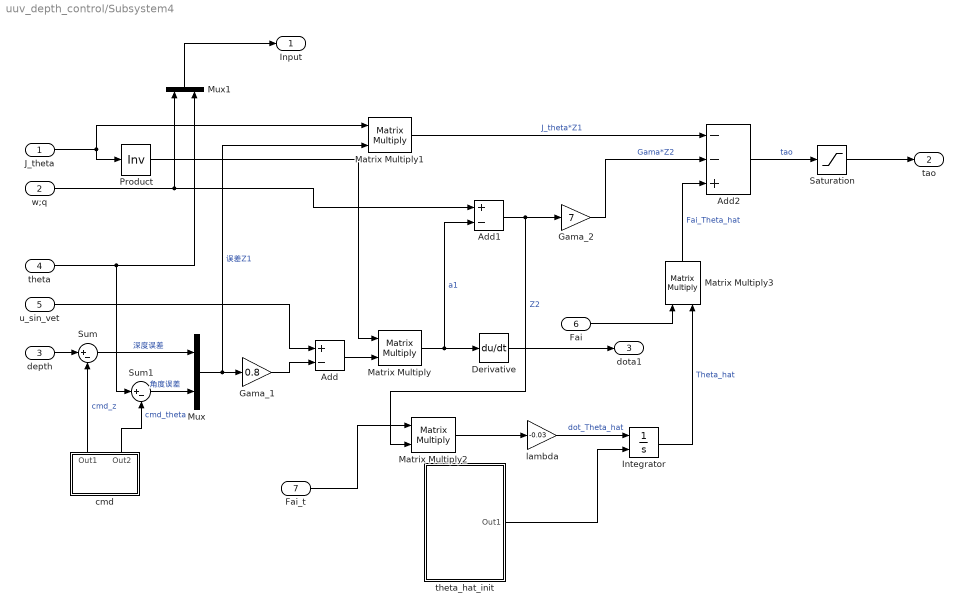
== system uuv_depth_control/Subsystem4 ==
  J_theta : Inport
  w;q : Inport  Port=2
  depth : Inport  Port=3
  theta : Inport  Port=4
  u_sin_vet : Inport  Port=5
  Fai : Inport  Port=6
  Fai_t : Inport  Port=7
  Add : Sum  Inputs=+-
  Add1 : Sum  Inputs=+-
  Add2 : Sum  Inputs=--+
  Derivative : Derivative
  Gama_1 : Gain  Gain=0.8
  Gama_2 : Gain  Gain=7
  Integrator : Integrator  InitialConditionSource=external
  Matrix Multiply{,1..3} (4 alike) : Product  Multiplication=Matrix(*)
  Mux : Mux  Inputs=2
  Mux1 : Mux  Inputs=2
  Product : Product  Inputs=/  Multiplication=Matrix(*)
  Saturation : Saturate  UpperLimit=120  LowerLimit=-100
  Sum : Sum  Inputs=|+-
  Sum1 : Sum  Inputs=|+-
  cmd : Subsystem
  lambda : Gain  Gain=-0.03
  theta_hat_init : Subsystem
  Input : Outport
  tao : Outport  Port=2
  dota1 : Outport  Port=3
  wires:
  Matrix Multiply/1 -> Add1/2, Derivative/1  "a1"
  Add2/1 -> Saturation/1  "tao"
  Add/1 -> Matrix Multiply/2
  cmd/1(Out1) -> Sum/2  "cmd_z"
  Add1/1 -> Gama_2/1, Matrix Multiply2/2  "Z2"
  Mux/1 -> Matrix Multiply1/2, Gama_1/1  "误差Z1"
  J_theta/1 -> Product/1, Matrix Multiply1/1
  Sum1/1 -> Mux/2  "角度误差"
  Gama_1/1 -> Add/2
  theta/1 -> Mux1/2, Sum1/1
  cmd/2(Out2) -> Sum1/2  "cmd_theta"
  Product/1 -> Matrix Multiply/1
  Matrix Multiply1/1 -> Add2/1  "J_theta*Z1"
  w;q/1 -> Add1/1, Mux1/1
  depth/1 -> Sum/1
  u_sin_vet/1 -> Add/1
  Mux1/1 -> Input/1
  Gama_2/1 -> Add2/2  "Gama*Z2"
  Matrix Multiply2/1 -> lambda/1
  Fai_t/1 -> Matrix Multiply2/1
  Fai/1 -> Matrix Multiply3/1
  Matrix Multiply3/1 -> Add2/3  "Fai_Theta_hat"
  Integrator/1 -> Matrix Multiply3/2  "Theta_hat"
  theta_hat_init/1(Out1) -> Integrator/2
  lambda/1 -> Integrator/1  "dot_Theta_hat"
  Derivative/1 -> dota1/1
  Sum/1 -> Mux/1  "深度误差"
  Saturation/1 -> tao/1

== system uuv_depth_control/speed_cintrol ==
  Input : Inport
  Abs2 : Abs
  Add1 : Sum  Inputs=-+
  Add3 : Sum
  Constant2 : Constant  Value=0.15
  Derivative2 : Derivative
  Integrator1 : Integrator
  Kinetic model : Subsystem
      settings: PortSchema="{\"entries\":[{\"content\":{\"sides\":[{\"content\":{\"connectorIds\":[\"In1\",\"In2\"]},\"type\":\"ConnectorPlacement.EquallySpacedRectSide\",\"uuid\":\"ab557843-e031-4248-b9d1-7c566f741c61\"},{\"content\":{\"connectorIds\":[\"Out1\",\"In3\"],\"side\":\"RIGHT\"},\"type\":\"ConnectorPlacement.EquallySpacedRectSide\",\"uuid\":\"21457043-a342-42ad-b992-fc1f26888830\"},{\"content\":{\"connectorIds\":[],\"side\":\"TOP\"},\"type\":\"ConnectorPlacement.EquallySpacedRectSide\",\"uuid\":\"46297411-6c48-4449-b379-31c60e59c869\"}]},\"type\":\"ConnectorPlacement.EquallySpacedConnector\",\"uuid\":\"5361bacf-5f38-4767-97c2-c3369bc5e695\"}],\"packageUris\":[\"http://schema.mathworks.com/mf0/Connector/R2020b\"],\"version\":\"1.0\"}"
  Matrix Multiply1 : Product  Multiplication=Matrix(*)
  Signal Generator1 : SignalGenerator  Amplitude=0.2  Frequency=0.0143
  Sum1 : Sum  Inputs=|++
  controller : Subsystem
  u : Outport
  wires:
  Integrator1/1 -> Kinetic model/3(Input), Add3/2, Matrix Multiply1/2, Abs2/1  "ur"
  Add1/1 -> controller/3(Z1)  "speed_error"
  Matrix Multiply1/1 -> controller/1(ur|ur|), Kinetic model/1(ur|ur|)  "ur|ur|"
  Kinetic model/1(dot_ur) -> Integrator1/1
  Add3/1 -> u/1, Add1/2  "u"
  Input/1 -> Add1/1, Derivative2/1  "ud"
  controller/1(tao_u) -> Kinetic model/2(tao_u)
  Abs2/1 -> Matrix Multiply1/1
  Derivative2/1 -> controller/2(dot_ud)  "dot_ud"
  Sum1/1 -> Add3/1  "uf"
  Constant2/1 -> Sum1/2
  Signal Generator1/1 -> Sum1/1

== system uuv_depth_control/speed_d ==
  Demux : Demux  Tag=STV Demux  Outputs=1
      settings: DisplayOption=none
  FromWs : FromWorkspace  Tag=STV FromWs  VariableName=tuvar
      SigBuilderData=|
      | common.afterFinalStr = 'Extrapolate'
      | common.sampleTime = 0
      | dataSet.timeRange = [0 10]
      | dataSet.name = 'Group 1'
      | sbobj.Groups.Name = 'Group 1'
      | sbobj.Groups.Signals.Name = 'Signal 1'
      | sbobj.Groups.Signals.XData = [0 10]
      | sbobj.Groups.Signals.YData = [1.2 1.2]
  Signal 1 : Outport  Tag=STV Outport
  wires:
  FromWs/1 -> Demux/1
  Demux/1 -> Signal 1/1

== system uuv_depth_control/动力学模型1 ==
  ur|ur| : Inport
  tao_u : Inport  Port=2
  Input : Inport  Port=3
  Add2 : Sum  Inputs=+++
  Constant5 : Constant  Value=-1
  Constant6 : Constant
  Divide : Product  Inputs=*/
  MATLAB Function : MATLAB Function  TreatAsAtomicUnit=on
  Matrix Multiply4 : Product  Multiplication=Matrix(*)
  Switch1 : Switch  Criteria=u2 > Threshold
  dot_ur : Outport
  wires:
  MATLAB Function/1(gama_true) -> Divide/2  "gama_true"
  MATLAB Function/2(beta_true) -> Matrix Multiply4/1  "beta_true"
  MATLAB Function/3(delta_true) -> Add2/3  "delta_true"
  Matrix Multiply4/1 -> Add2/2
  tao_u/1 -> Divide/1
  Divide/1 -> Add2/1
  Add2/1 -> dot_ur/1  "dot_ur"
  ur|ur|/1 -> Matrix Multiply4/2
  Input/1 -> Switch1/2
  Constant6/1 -> Switch1/1
  Constant5/1 -> Switch1/3
  Switch1/1 -> MATLAB Function/1(delta_u)  "delta_u"

== system uuv_depth_control/控制器 ==
  ur|ur| : Inport
  dot_ud : Inport  Port=2
  Z1 : Inport  Port=3
  Add : Sum  Inputs=----+
  Add4 : Sum  Inputs=+---+
  Constant1 : Constant  Value=-1
  Constant5 : Constant
  Gain : Gain  Gain=0.07
  Integrator4 : Integrator
  Integrator6 : Integrator  InitialCondition=-0.054
  Integrator7 : Integrator  InitialCondition=34.9
  Matrix Multiply{4,6..8} (4 alike) : Product  Multiplication=Matrix(*)
  Switch1 : Switch  Criteria=u2 > Threshold
  eta1 : Gain  Gain=0.01
  k1 : Gain  Gain=3
  tao_u : Outport
  wires:
  ur|ur|/1 -> Matrix Multiply4/1, Matrix Multiply7/1
  Constant1/1 -> Switch1/3
  Switch1/1 -> eta1/1
  Integrator7/1 -> Matrix Multiply8/2  "gama_hat"
  Constant5/1 -> Switch1/1
  Matrix Multiply7/1 -> Add/4, Add4/2  "beta_hat*ur|ur|"
  Integrator6/1 -> Matrix Multiply7/2  "beta_hat"
  Integrator4/1 -> Add/3, Add4/3  "dot_uf_hat"
  Add4/1 -> Matrix Multiply8/1
  k1/1 -> Add/2, Add4/4  "k1Z1"
  eta1/1 -> Add4/5, Add/1  "滑膜项"
  Gain/1 -> Matrix Multiply4/2, Matrix Multiply6/1, Integrator4/1  "dd_uf_hat"
  Matrix Multiply6/1 -> Integrator7/1  "dot_gama_hat"
  Matrix Multiply4/1 -> Integrator6/1  "dot_beta_hat"
  Add/1 -> Matrix Multiply6/2  "Fai"
  dot_ud/1 -> Add/5, Add4/1
  Matrix Multiply8/1 -> tao_u/1  "tao_u"
  Z1/1 -> Switch1/2, k1/1, Gain/1

== system uuv_depth_control/Subsystem/cmd ==
  Cmd Depth : Subsystem  Tag=STV Subsys  LoadFcn=sigbuilder_block('load');  StartFcn=sigbuilder_block('start');  StopFcn=sigbuilder_block('stop');  ClipboardFcn=sigbuilder_block('clipboard');  mask(Sigbuilder block){tuvar=[0:10]}
      mask help: Simulink:masks:SigbuilderBlock_MD
      mask init:
      | if ~strcmp(get_param(bdroot(gcbh),'SimulationStatus'),'stopped') tuvar = sigbuilder_block('maskInit'); end
      settings: CopyFcn=sigbuilder_block('copy');  DeleteFcn=sigbuilder_block('delete');  ModelCloseFcn=sigbuilder_block('modelClose');  PreSaveFcn=sigbuilder_block('preSave');  PauseFcn=sigbuilder_block('pause');  ContinueFcn=sigbuilder_block('continue');  NameChangeFcn=sigbuilder_block('namechange');  OpenFcn=sigbuilder_block('open',[238.2 69 550.8 375 ]);  CloseFcn=sigbuilder_block('close');
      mask Display: plot(0, 0, 100, 100,[2, 2, 32, 32, 2], [68, 8, 8, 68, 68],[32, 2], [38, 38], [32, 19, 2],[53, 60, 44], [32, 17, 17, 2],[16, 16, 31, 31]);txt = getActiveGroup(gcbh);text(2, 100, txt,'verticalAlignment', 'top');
  Cmd theta : Subsystem  Tag=STV Subsys  LoadFcn=sigbuilder_block('load');  StartFcn=sigbuilder_block('start');  StopFcn=sigbuilder_block('stop');  ClipboardFcn=sigbuilder_block('clipboard');  mask(Sigbuilder block){tuvar=[0:10]}
      mask help: Simulink:masks:SigbuilderBlock_MD
      mask init:
      | if ~strcmp(get_param(bdroot(gcbh),'SimulationStatus'),'stopped') tuvar = sigbuilder_block('maskInit'); end
      settings: CopyFcn=sigbuilder_block('copy');  DeleteFcn=sigbuilder_block('delete');  ModelCloseFcn=sigbuilder_block('modelClose');  PreSaveFcn=sigbuilder_block('preSave');  PauseFcn=sigbuilder_block('pause');  ContinueFcn=sigbuilder_block('continue');  NameChangeFcn=sigbuilder_block('namechange');  OpenFcn=sigbuilder_block('open',[589.2 96.6 550.8 400.8 ]);  CloseFcn=sigbuilder_block('close');
      mask Display: plot(0, 0, 100, 100,[2, 2, 32, 32, 2], [68, 8, 8, 68, 68],[32, 2], [38, 38], [32, 19, 2],[53, 60, 44], [32, 17, 17, 2],[16, 16, 31, 31]);txt = getActiveGroup(gcbh);text(2, 100, txt,'verticalAlignment', 'top');
  Out1 : Outport
  Out2 : Outport  Port=2
  wires:
  Cmd Depth/1(Signal 1) -> Out1/1  "cmd_z"
  Cmd theta/1(Signal 1) -> Out2/1  "cmd_theta"

== system uuv_depth_control/Subsystem1/cmd ==
  Cmd Depth : Subsystem  Tag=STV Subsys  LoadFcn=sigbuilder_block('load');  StartFcn=sigbuilder_block('start');  StopFcn=sigbuilder_block('stop');  ClipboardFcn=sigbuilder_block('clipboard');  mask(Sigbuilder block){tuvar=[0:10]}
      mask help: Simulink:masks:SigbuilderBlock_MD
      mask init:
      | if ~strcmp(get_param(bdroot(gcbh),'SimulationStatus'),'stopped') tuvar = sigbuilder_block('maskInit'); end
      settings: CopyFcn=sigbuilder_block('copy');  DeleteFcn=sigbuilder_block('delete');  ModelCloseFcn=sigbuilder_block('modelClose');  PreSaveFcn=sigbuilder_block('preSave');  PauseFcn=sigbuilder_block('pause');  ContinueFcn=sigbuilder_block('continue');  NameChangeFcn=sigbuilder_block('namechange');  OpenFcn=sigbuilder_block('open',[238.2 69 550.8 375 ]);  CloseFcn=sigbuilder_block('close');
      mask Display: plot(0, 0, 100, 100,[2, 2, 32, 32, 2], [68, 8, 8, 68, 68],[32, 2], [38, 38], [32, 19, 2],[53, 60, 44], [32, 17, 17, 2],[16, 16, 31, 31]);txt = getActiveGroup(gcbh);text(2, 100, txt,'verticalAlignment', 'top');
  Cmd theta : Subsystem  Tag=STV Subsys  LoadFcn=sigbuilder_block('load');  StartFcn=sigbuilder_block('start');  StopFcn=sigbuilder_block('stop');  ClipboardFcn=sigbuilder_block('clipboard');  mask(Sigbuilder block){tuvar=[0:10]}
      mask help: Simulink:masks:SigbuilderBlock_MD
      mask init:
      | if ~strcmp(get_param(bdroot(gcbh),'SimulationStatus'),'stopped') tuvar = sigbuilder_block('maskInit'); end
      settings: CopyFcn=sigbuilder_block('copy');  DeleteFcn=sigbuilder_block('delete');  ModelCloseFcn=sigbuilder_block('modelClose');  PreSaveFcn=sigbuilder_block('preSave');  PauseFcn=sigbuilder_block('pause');  ContinueFcn=sigbuilder_block('continue');  NameChangeFcn=sigbuilder_block('namechange');  OpenFcn=sigbuilder_block('open',[313.2 49.2 550.8 400.8 ]);  CloseFcn=sigbuilder_block('close');
      mask Display: plot(0, 0, 100, 100,[2, 2, 32, 32, 2], [68, 8, 8, 68, 68],[32, 2], [38, 38], [32, 19, 2],[53, 60, 44], [32, 17, 17, 2],[16, 16, 31, 31]);txt = getActiveGroup(gcbh);text(2, 100, txt,'verticalAlignment', 'top');
  Out1 : Outport
  Out2 : Outport  Port=2
  wires:
  Cmd Depth/1(Signal 1) -> Out1/1  "cmd_z"
  Cmd theta/1(Signal 1) -> Out2/1  "cmd_theta"

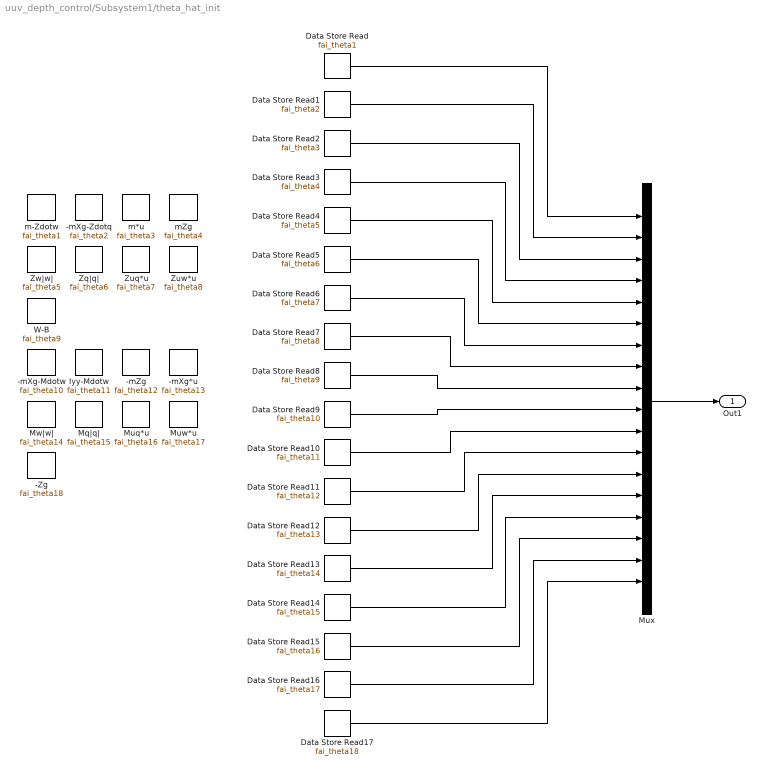
== system uuv_depth_control/Subsystem1/theta_hat_init ==
  -Zg : DataStoreMemory  DataStoreName=fai_theta18  ReadBeforeWriteMsg=warning  WriteAfterWriteMsg=warning  WriteAfterReadMsg=warning  InitialValue=-0.0196000000000000  ShowAdditionalParam=off
  -mXg*u : DataStoreMemory  DataStoreName=fai_theta13  ReadBeforeWriteMsg=warning  WriteAfterWriteMsg=warning  WriteAfterReadMsg=warning  ShowAdditionalParam=off
  -mXg-Mdotw : DataStoreMemory  DataStoreName=fai_theta10  ReadBeforeWriteMsg=warning  WriteAfterWriteMsg=warning  WriteAfterReadMsg=warning  InitialValue=1.93000000000000  ShowAdditionalParam=off
  -mXg-Zdotq : DataStoreMemory  DataStoreName=fai_theta2  ReadBeforeWriteMsg=warning  WriteAfterWriteMsg=warning  WriteAfterReadMsg=warning  InitialValue=1.930000000000000  ShowAdditionalParam=off
  -mZg : DataStoreMemory  DataStoreName=fai_theta12  ReadBeforeWriteMsg=warning  WriteAfterWriteMsg=warning  WriteAfterReadMsg=warning  InitialValue=-0.597408000000000  ShowAdditionalParam=off
  Data Store Read : DataStoreRead  DataStoreName=fai_theta1  IndexOptions=Index vector (dialog)  Indices=1  OutputSizes=1
  Data Store Read1 : DataStoreRead  DataStoreName=fai_theta2  IndexOptions=Index vector (dialog)  Indices=1  OutputSizes=1
  Data Store Read10 : DataStoreRead  DataStoreName=fai_theta11  IndexOptions=Index vector (dialog)  Indices=1  OutputSizes=1
  Data Store Read11 : DataStoreRead  DataStoreName=fai_theta12  IndexOptions=Index vector (dialog)  Indices=1  OutputSizes=1
  Data Store Read12 : DataStoreRead  DataStoreName=fai_theta13  IndexOptions=Index vector (dialog)  Indices=1  OutputSizes=1
  Data Store Read13 : DataStoreRead  DataStoreName=fai_theta14  IndexOptions=Index vector (dialog)  Indices=1  OutputSizes=1
  Data Store Read14 : DataStoreRead  DataStoreName=fai_theta15  IndexOptions=Index vector (dialog)  Indices=1  OutputSizes=1
  Data Store Read15 : DataStoreRead  DataStoreName=fai_theta16  IndexOptions=Index vector (dialog)  Indices=1  OutputSizes=1
  Data Store Read16 : DataStoreRead  DataStoreName=fai_theta17  IndexOptions=Index vector (dialog)  Indices=1  OutputSizes=1
  Data Store Read17 : DataStoreRead  DataStoreName=fai_theta18  IndexOptions=Index vector (dialog)  Indices=1  OutputSizes=1
  Data Store Read2 : DataStoreRead  DataStoreName=fai_theta3  IndexOptions=Index vector (dialog)  Indices=1  OutputSizes=1
  Data Store Read3 : DataStoreRead  DataStoreName=fai_theta4  IndexOptions=Index vector (dialog)  Indices=1  OutputSizes=1
  Data Store Read4 : DataStoreRead  DataStoreName=fai_theta5  IndexOptions=Index vector (dialog)  Indices=1  OutputSizes=1
  Data Store Read5 : DataStoreRead  DataStoreName=fai_theta6  IndexOptions=Index vector (dialog)  Indices=1  OutputSizes=1
  Data Store Read6 : DataStoreRead  DataStoreName=fai_theta7  IndexOptions=Index vector (dialog)  Indices=1  OutputSizes=1
  Data Store Read7 : DataStoreRead  DataStoreName=fai_theta8  IndexOptions=Index vector (dialog)  Indices=1  OutputSizes=1
  Data Store Read8 : DataStoreRead  DataStoreName=fai_theta9  IndexOptions=Index vector (dialog)  Indices=1  OutputSizes=1
  Data Store Read9 : DataStoreRead  DataStoreName=fai_theta10  IndexOptions=Index vector (dialog)  Indices=1  OutputSizes=1
  Iyy-Mdotw : DataStoreMemory  DataStoreName=fai_theta11  ReadBeforeWriteMsg=warning  WriteAfterWriteMsg=warning  WriteAfterReadMsg=warning  InitialValue=8.330000000000000  ShowAdditionalParam=off
  Mq|q| : DataStoreMemory  DataStoreName=fai_theta15  ReadBeforeWriteMsg=warning  WriteAfterWriteMsg=warning  WriteAfterReadMsg=warning  InitialValue=-9.40000000000000  ShowAdditionalParam=off
  Muq*u : DataStoreMemory  DataStoreName=fai_theta16  ReadBeforeWriteMsg=warning  WriteAfterWriteMsg=warning  WriteAfterReadMsg=warning  InitialValue=-1  ShowAdditionalParam=off
  Muw*u : DataStoreMemory  DataStoreName=fai_theta17  ReadBeforeWriteMsg=warning  WriteAfterWriteMsg=warning  WriteAfterReadMsg=warning  InitialValue=12  ShowAdditionalParam=off
  Mux : Mux  Inputs=18
  Mw|w| : DataStoreMemory  DataStoreName=fai_theta14  ReadBeforeWriteMsg=warning  WriteAfterWriteMsg=warning  WriteAfterReadMsg=warning  InitialValue=3.18000000000000  ShowAdditionalParam=off
  W-B : DataStoreMemory  DataStoreName=fai_theta9  ReadBeforeWriteMsg=warning  WriteAfterWriteMsg=warning  WriteAfterReadMsg=warning  InitialValue=-9  ShowAdditionalParam=off
  Zq|q| : DataStoreMemory  DataStoreName=fai_theta6  ReadBeforeWriteMsg=warning  WriteAfterWriteMsg=warning  WriteAfterReadMsg=warning  InitialValue=-0.632000000000000  ShowAdditionalParam=off
  Zuq*u : DataStoreMemory  DataStoreName=fai_theta7  ReadBeforeWriteMsg=warning  WriteAfterWriteMsg=warning  WriteAfterReadMsg=warning  InitialValue=-2.61000000000000  ShowAdditionalParam=off
  Zuw*u : DataStoreMemory  DataStoreName=fai_theta8  ReadBeforeWriteMsg=warning  WriteAfterWriteMsg=warning  WriteAfterReadMsg=warning  InitialValue=-14.3000000000000  ShowAdditionalParam=off
  Zw|w| : DataStoreMemory  DataStoreName=fai_theta5  ReadBeforeWriteMsg=warning  WriteAfterWriteMsg=warning  WriteAfterReadMsg=warning  InitialValue=-131  ShowAdditionalParam=off
  m*u : DataStoreMemory  DataStoreName=fai_theta3  ReadBeforeWriteMsg=warning  WriteAfterWriteMsg=warning  WriteAfterReadMsg=warning  InitialValue=15.2400000000000  ShowAdditionalParam=off
  m-Zdotw : DataStoreMemory  DataStoreName=fai_theta1  ReadBeforeWriteMsg=warning  WriteAfterWriteMsg=warning  WriteAfterReadMsg=warning  InitialValue=65.980000000000000  ShowAdditionalParam=off
  mZg : DataStoreMemory  DataStoreName=fai_theta4  ReadBeforeWriteMsg=warning  WriteAfterWriteMsg=warning  WriteAfterReadMsg=warning  InitialValue=0.597408000000000  ShowAdditionalParam=off
  Out1 : Outport
  wires:
  Mux/1 -> Out1/1
  Data Store Read/1 -> Mux/1
  Data Store Read3/1 -> Mux/4
  Data Store Read8/1 -> Mux/9
  Data Store Read5/1 -> Mux/6
  Data Store Read10/1 -> Mux/11
  Data Store Read4/1 -> Mux/5
  Data Store Read15/1 -> Mux/16
  Data Store Read12/1 -> Mux/13
  Data Store Read1/1 -> Mux/2
  Data Store Read14/1 -> Mux/15
  Data Store Read9/1 -> Mux/10
  Data Store Read7/1 -> Mux/8
  Data Store Read13/1 -> Mux/14
  Data Store Read2/1 -> Mux/3
  Data Store Read6/1 -> Mux/7
  Data Store Read17/1 -> Mux/18
  Data Store Read11/1 -> Mux/12
  Data Store Read16/1 -> Mux/17

== system uuv_depth_control/Subsystem2/cmd ==
  Add : Sum
  Cmd Depth : Subsystem  Tag=STV Subsys  LoadFcn=sigbuilder_block('load');  StartFcn=sigbuilder_block('start');  StopFcn=sigbuilder_block('stop');  ClipboardFcn=sigbuilder_block('clipboard');  mask(Sigbuilder block){tuvar=[0:10]}
      mask help: Simulink:masks:SigbuilderBlock_MD
      mask init:
      | if ~strcmp(get_param(bdroot(gcbh),'SimulationStatus'),'stopped') tuvar = sigbuilder_block('maskInit'); end
      settings: CopyFcn=sigbuilder_block('copy');  DeleteFcn=sigbuilder_block('delete');  ModelCloseFcn=sigbuilder_block('modelClose');  PreSaveFcn=sigbuilder_block('preSave');  PauseFcn=sigbuilder_block('pause');  ContinueFcn=sigbuilder_block('continue');  NameChangeFcn=sigbuilder_block('namechange');  OpenFcn=sigbuilder_block('open',[361.8 75 550.8 375 ]);  CloseFcn=sigbuilder_block('close');
      mask Display: plot(0, 0, 100, 100,[2, 2, 32, 32, 2], [68, 8, 8, 68, 68],[32, 2], [38, 38], [32, 19, 2],[53, 60, 44], [32, 17, 17, 2],[16, 16, 31, 31]);txt = getActiveGroup(gcbh);text(2, 100, txt,'verticalAlignment', 'top');
  Cmd theta : Subsystem  Tag=STV Subsys  LoadFcn=sigbuilder_block('load');  StartFcn=sigbuilder_block('start');  StopFcn=sigbuilder_block('stop');  ClipboardFcn=sigbuilder_block('clipboard');  mask(Sigbuilder block){tuvar=[0:10]}
      mask help: Simulink:masks:SigbuilderBlock_MD
      mask init:
      | if ~strcmp(get_param(bdroot(gcbh),'SimulationStatus'),'stopped') tuvar = sigbuilder_block('maskInit'); end
      settings: CopyFcn=sigbuilder_block('copy');  DeleteFcn=sigbuilder_block('delete');  ModelCloseFcn=sigbuilder_block('modelClose');  PreSaveFcn=sigbuilder_block('preSave');  PauseFcn=sigbuilder_block('pause');  ContinueFcn=sigbuilder_block('continue');  NameChangeFcn=sigbuilder_block('namechange');  OpenFcn=sigbuilder_block('open',[313.2 49.2 550.8 400.8 ]);  CloseFcn=sigbuilder_block('close');
      mask Display: plot(0, 0, 100, 100,[2, 2, 32, 32, 2], [68, 8, 8, 68, 68],[32, 2], [38, 38], [32, 19, 2],[53, 60, 44], [32, 17, 17, 2],[16, 16, 31, 31]);txt = getActiveGroup(gcbh);text(2, 100, txt,'verticalAlignment', 'top');
  Constant1 : Constant  Value=-1
  Constant2 : Constant  Value=0
  Constant3 : Constant
  Constant4 : Constant  Value=0
  Signal Generator : SignalGenerator  Amplitude=3  Frequency=0.1  Units=rad/sec
  Switch : Switch  Criteria=u2 > Threshold
  Switch1 : Switch  Criteria=u2 > Threshold
  Out1 : Outport
  Out2 : Outport  Port=2
  wires:
  Cmd Depth/1(Signal 2) -> Add/2
  Cmd theta/1(Signal 1) -> Switch1/1
  Signal Generator/1 -> Switch/1
  Add/1 -> Out1/1  "cmd_z"
  Constant4/1 -> Switch/3
  Switch/1 -> Add/1
  Constant1/1 -> Switch/2
  Constant2/1 -> Switch1/3
  Constant3/1 -> Switch1/2
  Switch1/1 -> Out2/1  "cmd_theta"
